simulink model "MP_H"  (R2019a)
settings: Solver=VariableStepAuto  StartTime=0.0  StopTime=10.0  RelTol=1e-3
undefined symbols (not defined in the file): Fx0, Fy0, kd, kp, N, tau_BP, tau_PN, ThetaA_cst, ThetaE_cst, thetaP_init, Ts
libraries: dspsigops x4
settings Model: Creator=leand  LastModifiedBy=leand

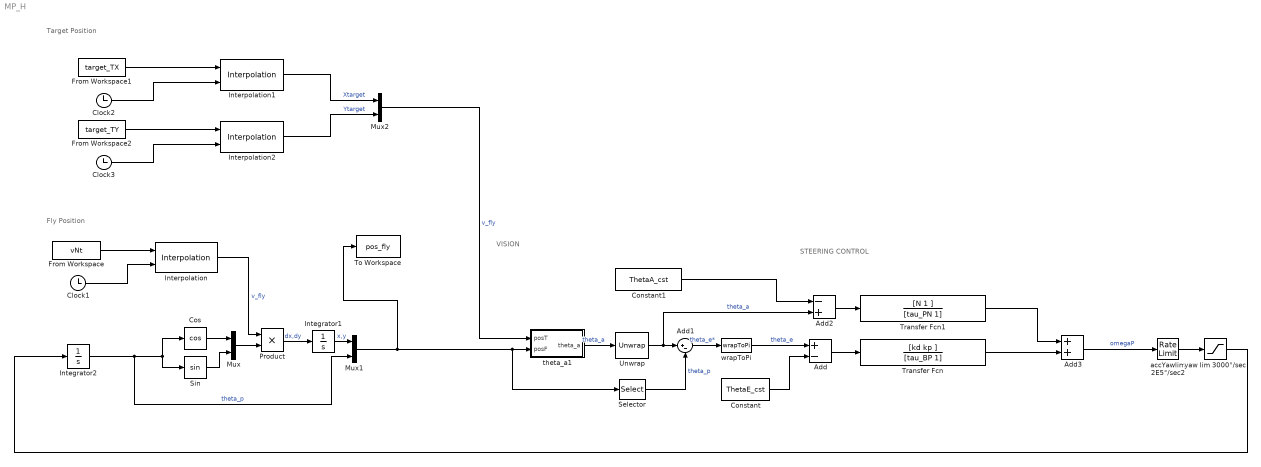
== system MP_H ==
  note: VISION
  note: STEERING CONTROL
  note: Target Position
  note: Fly Position
  Add : Sum  Inputs=+-
  Add1 : Sum  Inputs=|+-
  Add2 : Sum  Inputs=-+
  Add3 : Sum
  Clock1 : Clock
  Clock2 : Clock
  Clock3 : Clock
  Constant : Constant  Value=ThetaE_cst
  Constant1 : Constant  Value=ThetaA_cst
  Cos : Trigonometry  Operator=cos
  From Workspace : FromWorkspace  VariableName=vNt  SampleTime=0
  From Workspace1 : FromWorkspace  VariableName=target_TX  SampleTime=0
  From Workspace2 : FromWorkspace  VariableName=target_TY  SampleTime=0
  Integrator1 : Integrator  InitialCondition=[Fx0 Fy0]
  Integrator2 : Integrator  InitialCondition=thetaP_init
  Interpolation : dspsigops/Interpolation  InterpSource=Input port  InterpPoints=[1.1 4.8 2.67 1.6 3.2]'  InterpMode=Linear  InterpL=3  InterpR=3  InterpAlpha=0.5  InvalidMode=Clip
      settings: SourceProductName=DSP System Toolbox  SourceProductBaseCode=DS
  Interpolation1 : dspsigops/Interpolation  InterpSource=Input port  InterpPoints=[1.1 4.8 2.67 1.6 3.2]'  InterpMode=Linear  InterpL=3  InterpR=3  InterpAlpha=0.5  InvalidMode=Clip
      settings: SourceProductName=DSP System Toolbox  SourceProductBaseCode=DS
  Interpolation2 : dspsigops/Interpolation  InterpSource=Input port  InterpPoints=[1.1 4.8 2.67 1.6 3.2]'  InterpMode=Linear  InterpL=3  InterpR=3  InterpAlpha=0.5  InvalidMode=Clip
      settings: SourceProductName=DSP System Toolbox  SourceProductBaseCode=DS
  Mux : Mux  Inputs=2
  Mux1 : Mux  Inputs=2
  Mux2 : Mux  Inputs=2
  Product : Product
  Selector : Selector  InputPortWidth=3  IndexOptions=Index vector (dialog)  Indices=[3]  OutputSizes=1
  Sin : Trigonometry
  To Workspace : ToWorkspace  VariableName=pos_fly  SampleTime=Ts
  Transfer Fcn : TransferFcn  Numerator=[kd kp ]  Denominator=[tau_BP 1]
  Transfer Fcn1 : TransferFcn  Numerator=[N 1 ]  Denominator=[tau_PN 1]
  Unwrap : dspsigops/Unwrap  tol=pi  InputProcessing=Columns as channels (frame based)  running=off
  accYawlim 2E5°/sec2 : RateLimiter  RisingSlewLimit=deg2rad(2E5)  FallingSlewLimit=-deg2rad(2E5)  SampleTimeMode=inherited
  theta_a1 : MATLAB Function  TreatAsAtomicUnit=on
  wrapToPi : MATLABFcn  MATLABFcn=wrapToPi
  yaw lim 3000°/sec : Saturate  UpperLimit=deg2rad(3000)  LowerLimit=-deg2rad(3000)
  wires:
  theta_a1/1(theta_a) -> Unwrap/1  "theta_a"
  Add/1 -> Transfer Fcn/1
  Add1/1 -> wrapToPi/1  "theta_e*"
  Unwrap/1 -> Add2/2, Add1/1  "theta_a"
  Selector/1 -> Add1/2  "theta_p"
  wrapToPi/1 -> Add/1  "theta_e"
  Constant/1 -> Add/2
  Add2/1 -> Transfer Fcn1/1
  Constant1/1 -> Add2/1
  Transfer Fcn1/1 -> Add3/1
  Transfer Fcn/1 -> Add3/2
  Clock2/1 -> Interpolation1/2
  From Workspace2/1 -> Interpolation2/1
  From Workspace/1 -> Interpolation/1
  Interpolation/1 -> Product/1  "v_fly"
  Mux/1 -> Product/2
  Clock3/1 -> Interpolation2/2
  Clock1/1 -> Interpolation/2
  Cos/1 -> Mux/1
  Integrator1/1 -> Mux1/1  "x,y"
  Sin/1 -> Mux/2
  From Workspace1/1 -> Interpolation1/1
  Mux1/1 -> Selector/1, theta_a1/2(posF), To Workspace/1
  Interpolation1/1 -> Mux2/1  "Xtarget"
  Integrator2/1 -> Mux1/2, Cos/1, Sin/1  "theta_p"
  Mux2/1 -> theta_a1/1(posT)  "v_fly"
  Product/1 -> Integrator1/1  "dx,dy"
  Interpolation2/1 -> Mux2/2  "Ytarget"
  Add3/1 -> accYawlim 2E5°/sec2/1  "omegaP"
  accYawlim 2E5°/sec2/1 -> yaw lim 3000°/sec/1
  yaw lim 3000°/sec/1 -> Integrator2/1

== matlab function MP_H/theta_a1 ==
  data: posT input; posF input; theta_a output
function theta_a  = fcn( posT, posF)

% theta_a = cart2pol(posT(1),posT(2));
% theta_p = cart2pol(posF(1),posF(2));
% theta_e = angdiff(theta_a,theta_p);

theta_a = atan2(posT(2)-posF(2),posT(1)-posF(1));
% if theta_a <=0
% theta_a = theta_a + 2*pi;
% end
% if posT(2)<=posF(2)
% theta_a = theta_a +2*pi;
% end

% theta_a = unwrap(theta_a);

end
